simulink model "generate_cartesian_velocity_motion"  (R2023a)
settings: Solver=FixedStepDiscrete  StartTime=0.0  StopTime=inf  FixedStep=0.001  RelTol=1e-3  EnableMultiTasking=on
PreLoadFcn:
  | frs = FrankaRobotSettings();
libraries: simulink x3, franka_simulink_library x2
settings Model: SimulationMode=external  ExtModeTrigDuration=10000  Creator=vasi_ko  LastModifiedBy=kvasios
settings SolverCC: AlgebraicLoopSolver=TrustRegion
settings DataIOCC: LimitDataPoints=on  SaveFormat=Array  ReturnWorkspaceOutputs=off
settings OptimizationCC: DefaultParameterBehavior=Inlined  EnhancedBackFolding=on  PassReuseOutputArgsThreshold=0  OptimizeBlockOrder=speed  DifferentSizesBufferReuse=on  OptimizationCustomize=off
settings DebuggingCC: SolverPrmCheckMsg=warning  ParameterTunabilityLossMsg=error  UnconnectedInputMsg=warning  UnconnectedOutputMsg=warning  UnconnectedLineMsg=warning  SFUnexpectedBacktrackingDiag=warning  SFNoUnconditionalDefaultTransitionDiag=warning  SFExecutionAtInitializationDiag=none  ArithmeticOperatorsInVariantConditions=warning
settings ModelReferenceCC: EnableRefExpFcnMdlSchedulingChecks=on  PropagateSignalLabelsOutOfModel=off
settings SFSimCC: SimUseLocalCustomCode=off  MATLABDynamicMemAlloc=off  CustomCodeUndefinedFunction=UseInterfaceOnly  SimTargetLang=C++
settings RTWCC: RTWVerbose=off  RTWUseLocalCustomCode=off  BuildConfiguration=Faster Runs  TargetLang=C++  DLArmComputeVersion=19.05
settings CodeAppCC: ForceParamTrailComments=on  OperatorAnnotations=on
settings ConfigComp: CovMetricSettings=dw  CovSaveCumulativeToWorkspaceVar=on  CovSaveSingleToWorkspaceVar=on  CovExternalEMLEnable=off  CovSFcnEnable=off

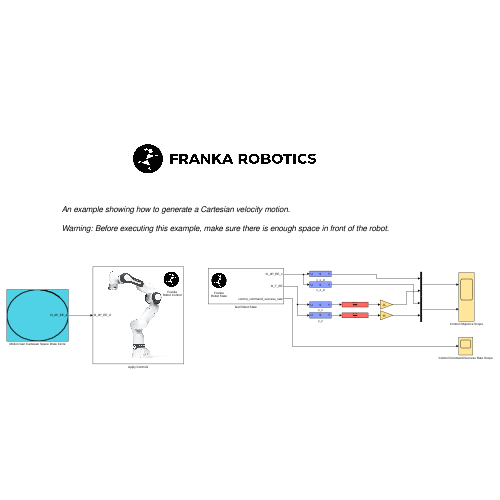
[thumbnail: Simulink's stored preview of the top-level diagram]
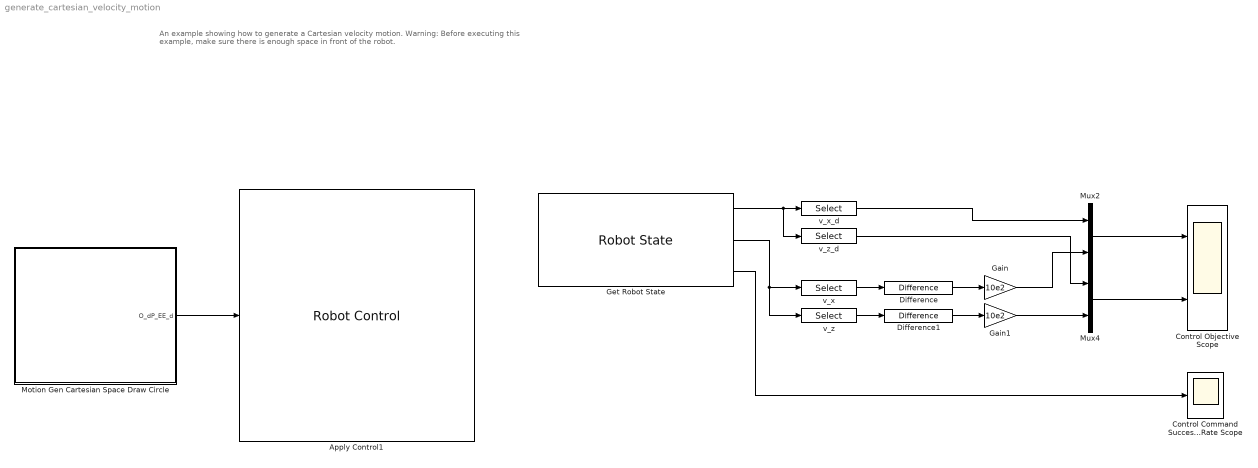
== system generate_cartesian_velocity_motion ==
  note: An example showing how to generate a Cartesian velocity motion.
      |
      | Warning: Before executing this example, make sure there is enough space in front of the robot.
  Apply Control1 : franka_simulink_library/Robot Control  robot_ip=frs.robot_ip  gripper_selection=None  control_mode=Cartesian Velocities - Internal Controller Mode  controller_choice=Joint Impedance Controller  joint_impedance=frs.joint_impedance_stiffness  cartesian_impedance=[3000, 3000, 3000, 300, 300, 300]  rate_limiter=on  cuttoff_frequency=frs.cutoff_frequency  elbow_control=off  collision_thresholds=[25 25 22 20 19 17 14 35 35 32 30 29 27 24 25 25 22 20 19 17 14 35 35 32 30 29 27 24 30 30 30 25 25 25 40 40 40 35 35 35 30 30 30 25 25 25 40 40 40 35 35 35]  load_inertia=frs.load_inertia.getAs1DArray  NE_T_EE=frs.NE_T_EE(:)  EE_T_K=frs.EE_T_K(:)  init_joint_configuration_req=on  init_joint_configuration=frs.home_configuration
      settings: SourceProductName=Franka Robotics Simulink Support Package
  Control Command Success Rate Scope : Scope
  Control Objective Scope : Scope  NumInputPorts=2
  Difference : simulink/Discrete/Difference  ICPrevInput=0.3069  OutMin=[]  OutMax=[]  OutDataType=fixdt(1, 16)  OutScaling=2^-10  DoSatur=off
  Difference1 : simulink/Discrete/Difference  ICPrevInput=0.5902  OutMin=[]  OutMax=[]  OutDataType=fixdt(1, 16)  OutScaling=2^-10  DoSatur=off
  Gain : Gain  Gain=10e2
  Gain1 : Gain  Gain=10e2
  Get Robot State : franka_simulink_library/Robot State  robot_ip=frs.robot_ip  signals_requested='O_dP_EE_c O_T_EE control_command_success_rate'
      settings: SourceProductName=Franka Robotics Simulink Support Package
  Motion Gen Cartesian Space Draw Circle : Subsystem
      mask Display:
      | pos = get_param(gcb, 'Position');
      | width = pos(3) - pos(1);
      | x = [0:width];
      | y = sin(x/180*pi);
      | % Parameters 'm' and 'b' must be defined in 'Parameters & Dialog' pane.
      | plot((1/2)*cos(x/180*2*pi+pi/4), (1/2)*sin(x/180*2*pi+pi/4));
      | 
      | port_label('output',1,'O_dP_EE_d');
  Mux2 : Mux  Inputs=2
  Mux4 : Mux  Inputs=2
  v_x : Selector  InputPortWidth=16  IndexOptions=Index vector (dialog)  Indices=13  OutputSizes=1
  v_x_d : Selector  InputPortWidth=6  IndexOptions=Index vector (dialog)  Indices=1  OutputSizes=1
  v_z : Selector  InputPortWidth=16  IndexOptions=Index vector (dialog)  Indices=15  OutputSizes=1
  v_z_d : Selector  InputPortWidth=6  IndexOptions=Index vector (dialog)  Indices=3  OutputSizes=1
  wires:
  Motion Gen Cartesian Space Draw Circle/1(O_dP_EE_d) -> Apply Control1/1
  Get Robot State/1 -> v_z_d/1, v_x_d/1
  Get Robot State/2 -> v_z/1, v_x/1
  v_x/1 -> Difference/1
  v_z/1 -> Difference1/1
  Difference/1 -> Gain/1
  Difference1/1 -> Gain1/1
  Gain1/1 -> Mux4/2
  Gain/1 -> Mux2/2
  v_x_d/1 -> Mux2/1
  v_z_d/1 -> Mux4/1
  Mux2/1 -> Control Objective Scope/1
  Mux4/1 -> Control Objective Scope/2
  Get Robot State/3 -> Control Command Success Rate Scope/1

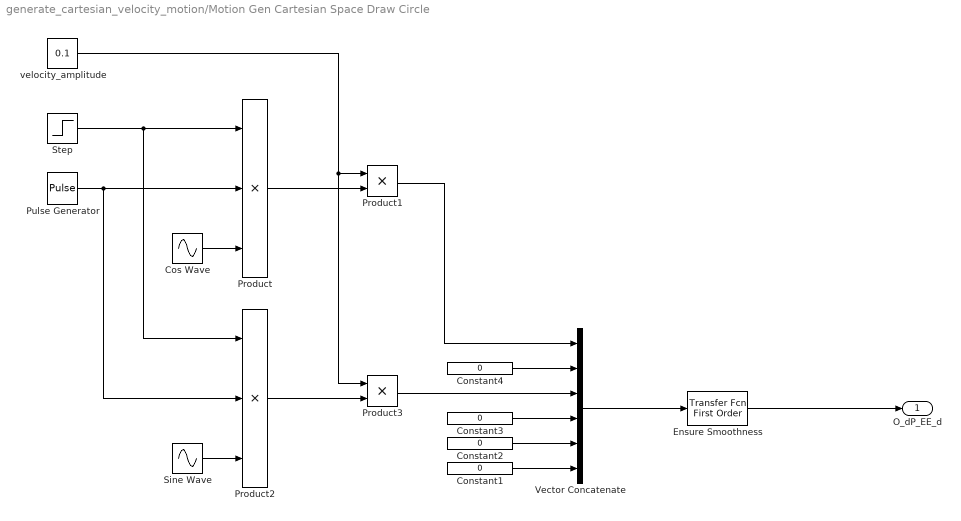
== system generate_cartesian_velocity_motion/Motion Gen Cartesian Space Draw Circle ==
  Constant{1..4} (4 alike) : Constant  Value=0  VectorParams1D=off
  Cos Wave : Sin  Frequency=pi  Phase=pi+pi/2  SampleTime=0
  Ensure Smoothness : simulink/Discrete/Transfer Fcn First Order  PoleZ=0.99  ICPrevOutput=0.0  DoSatur=off
  Product : Product  Inputs=3
  Product1 : Product
  Product2 : Product  Inputs=3
  Product3 : Product
  Pulse Generator : DiscretePulseGenerator  PulseType=Time based  Period=20  PulseWidth=50  PhaseDelay=1
  Sine Wave : Sin  Frequency=pi  Phase=pi  SampleTime=0
  Step : Step  Time=9  Before=1  After=0  SampleTime=0
  Vector Concatenate : Concatenate  NumInputs=6
  velocity_amplitude : Constant  Value=0.1  VectorParams1D=off
  O_dP_EE_d : Outport  VectorParamsAs1DForOutWhenUnconnected=off
  wires:
  Product1/1 -> Vector Concatenate/1
  Product3/1 -> Vector Concatenate/3
  Product2/1 -> Product3/2
  Sine Wave/1 -> Product2/3
  Pulse Generator/1 -> Product/2, Product2/2
  Step/1 -> Product/1, Product2/1
  velocity_amplitude/1 -> Product1/1, Product3/1
  Constant4/1 -> Vector Concatenate/2
  Constant3/1 -> Vector Concatenate/4
  Constant2/1 -> Vector Concatenate/5
  Constant1/1 -> Vector Concatenate/6
  Vector Concatenate/1 -> Ensure Smoothness/1
  Product/1 -> Product1/2
  Cos Wave/1 -> Product/3
  Ensure Smoothness/1 -> O_dP_EE_d/1
